simulink model "p3_car"  (R2025b)
settings: Solver=ode5  StartTime=0.0  StopTime=765  FixedStep=0.001  RelTol=1e-3
values from neighbouring files (symbols this model uses):
  DriveData = [ ... (first row only)    [fueleconomyinit.m]    (also in initDriveCycle.m; urbandrivinginit.m)
  Time = (0:1:765)'    [fueleconomyinit.m]    (also in initDriveCycle.m; urbandrivinginit.m = (0:1:1369)')
undefined symbols (not defined in the file or in its folder): datCar
settings Model: Creator=dxego  LastModifiedBy=ianw
settings OptimizationCC: ReuseModelBlockBuffer=off
settings DebuggingCC: AlgebraicLoopMsg=none
settings RTWCC: GPUComputeCapability=3.5

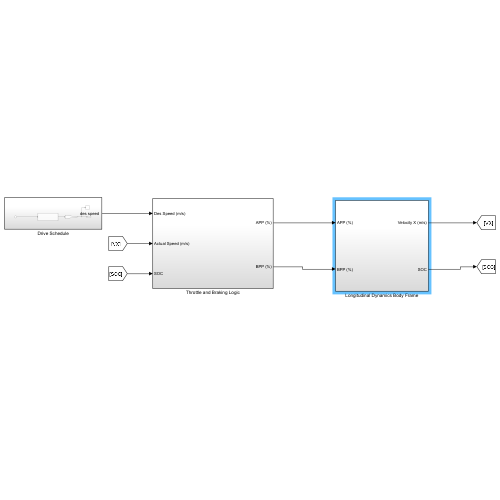
[thumbnail: Simulink's stored preview of the top-level diagram]
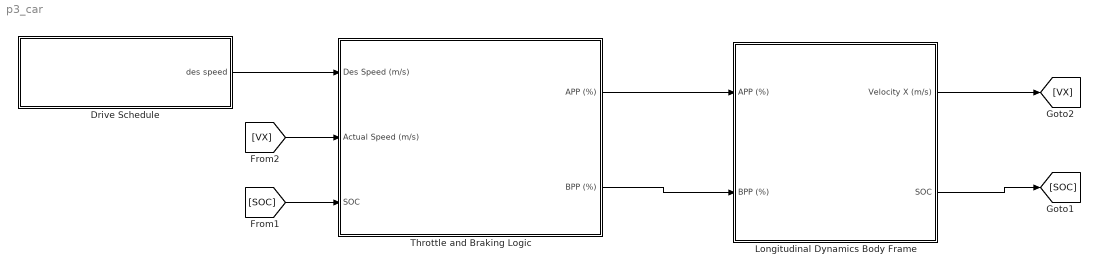
== system p3_car ==
  Drive Schedule : Subsystem
  Longitudinal Dynamics Body Frame : Subsystem
  "Throttle and Braking Logic " : Subsystem
  wires:
  "Throttle and Braking Logic "/1(APP (%)) -> Longitudinal Dynamics Body Frame/1(APP (%))
  "Throttle and Braking Logic "/2(BPP (%)) -> Longitudinal Dynamics Body Frame/2("BPP (%) ")
  Longitudinal Dynamics Body Frame/1(Velocity X (m/s)) -> [VX]
  Drive Schedule/1("des speed ") -> "Throttle and Braking Logic "/1("Des Speed (m/s) ")
  Longitudinal Dynamics Body Frame/2(SOC) -> [SOC]
  [SOC] -> "Throttle and Braking Logic "/3(SOC)
  [VX] -> "Throttle and Braking Logic "/2(Actual Speed (m/s))

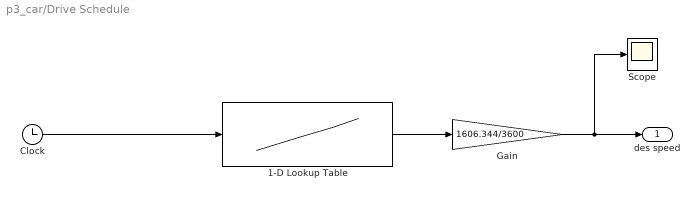
== system p3_car/Drive Schedule ==
  1-D Lookup Table : Lookup_n-D  NumberOfTableDimensions=1  BreakpointsForDimension1=Time  Table=DriveData  InternalRulePriority=Speed  RndMeth=Simplest
  Clock : Clock
  Gain : Gain  Gain=1606.344/3600
  Scope : Scope
      settings: ActiveDisplayYMinimum=-3.15  ActiveDisplayYMaximum=28.35  DataLoggingVariableName=ScopeData4
  "des speed " : Outport  VectorParamsAs1DForOutWhenUnconnected=off
  wires:
  Clock/1 -> 1-D Lookup Table/1
  1-D Lookup Table/1 -> Gain/1
  Gain/1 -> Scope/1, "des speed "/1

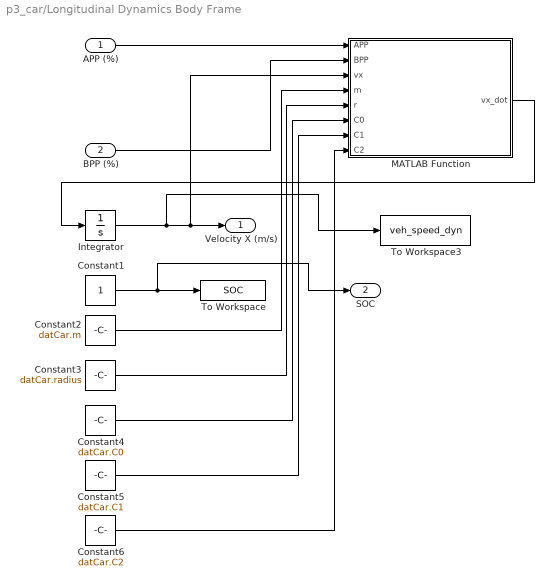
== system p3_car/Longitudinal Dynamics Body Frame ==
  APP (%) : Inport
  "BPP (%) " : Inport  Port=2
  Constant1 : Constant
  Constant2 : Constant  Value=datCar.m
  Constant3 : Constant  Value=datCar.radius
  Constant4 : Constant  Value=datCar.C0
  Constant5 : Constant  Value=datCar.C1
  Constant6 : Constant  Value=datCar.C2
  Integrator : Integrator  InitialCondition=datCar.init.vx0
  MATLAB Function : MATLAB Function  TreatAsAtomicUnit=on
  To Workspace : ToWorkspace  VariableName=SOC  SaveFormat=Timeseries  SampleTime=-1
  To Workspace3 : ToWorkspace  VariableName=veh_speed_dyn  SaveFormat=Timeseries  SampleTime=-1
  Velocity X (m/s) : Outport
  SOC : Outport  Port=2
  wires:
  APP (%)/1 -> MATLAB Function/1(APP)
  "BPP (%) "/1 -> MATLAB Function/2(BPP)
  Integrator/1 -> To Workspace3/1, Velocity X (m/s)/1, MATLAB Function/3(vx)
  Constant1/1 -> SOC/1, To Workspace/1
  MATLAB Function/1(vx_dot) -> Integrator/1
  Constant2/1 -> MATLAB Function/4(m)
  Constant3/1 -> MATLAB Function/5(r)
  Constant4/1 -> MATLAB Function/6(C0)
  Constant5/1 -> MATLAB Function/7(C1)
  Constant6/1 -> MATLAB Function/8(C2)

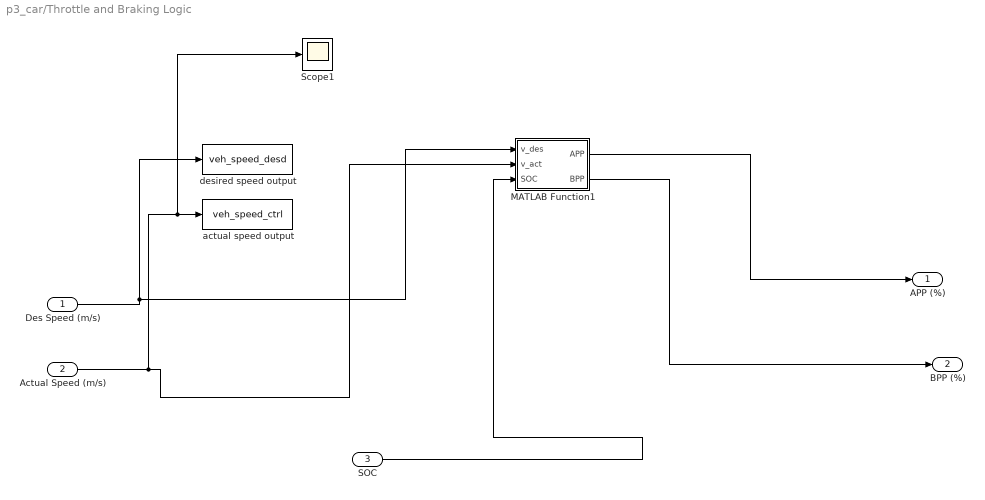
== system p3_car/Throttle and Braking Logic  ==
  "Des Speed (m/s) " : Inport
  Actual Speed (m/s) : Inport  Port=2
  SOC : Inport  Port=3
  MATLAB Function1 : MATLAB Function  TreatAsAtomicUnit=on
  Scope1 : Scope
      settings: ActiveDisplayYMinimum=-3.08288  ActiveDisplayYMaximum=27.75461
  actual speed output : ToWorkspace  VariableName=veh_speed_ctrl  SaveFormat=Timeseries  SampleTime=-1
  desired speed output : ToWorkspace  VariableName=veh_speed_desd  SaveFormat=Timeseries  SampleTime=-1
  APP (%) : Outport
  BPP (%) : Outport  Port=2
  wires:
  Actual Speed (m/s)/1 -> Scope1/1, actual speed output/1, MATLAB Function1/2(v_act)
  "Des Speed (m/s) "/1 -> MATLAB Function1/1(v_des), desired speed output/1
  SOC/1 -> MATLAB Function1/3(SOC)
  MATLAB Function1/1(APP) -> APP (%)/1
  MATLAB Function1/2(BPP) -> BPP (%)/1

== matlab function p3_car/Longitudinal Dynamics Body Frame/MATLAB Function ==
  data: APP input; vx_dot output; BPP input; vx input; m input; r input; C0 input; C1 input; C2 input
function vx_dot = fcn(APP,BPP,vx,m,r,C0,C1,C2)
%#codegen

vx_dot = 0;

T_drive_max = 4500;
T_brake_max = 7000;

T_drive = (APP/100) * T_drive_max;
T_brake = (BPP/100) * T_brake_max;

F_drive = T_drive / r;
F_brake = T_brake / r;
F_drag = C0 + C1*vx + C2*vx^2;

vx_dot = (F_drive - F_brake - F_drag) / m;

== matlab function p3_car/Throttle and Braking Logic /MATLAB Function1 ==
  data: v_des input; APP output; v_act input; SOC input; BPP output
function [APP,BPP] = fcn(v_des,v_act,SOC)
%#codegen

e = v_des - v_act;

Kp_throttle = 15;
Kp_brake = 20;

APP = 0;
BPP = 0;

if e >= 0
    APP = Kp_throttle * e;
    BPP = 0;
else
    APP = 0;
    BPP = Kp_brake * (-e);
end

APP = min(max(APP,0),100);
BPP = min(max(BPP,0),100);
